simulink model "test_lqi"  (R2018b)
settings: Solver=VariableStepAuto  StartTime=0.0  StopTime=50  RelTol=1e-3
values from neighbouring files (symbols this model uses):
  A = [ 0 0 1 0 ... (first row only)    [ControlParameters.m]    (also in FrutaFuruta.m; furutadynamics.m)
  B1 = [0; 0 ; b31 ; b41]/1000    [ControlParameters.m]    (also in FrutaFuruta.m; furutadynamics.m)
  C = [ 1 0 0 0]    [ControlParameters.m]    (also in FrutaFuruta.m; furutadynamics.m)
  ki = K(5)    [ControlParameters.m]    (also in FrutaFuruta.m; furutadynamics.m)
undefined symbols (not defined in the file or in its folder): K1
settings Model: Creator=Jones  LastModifiedBy=Jones

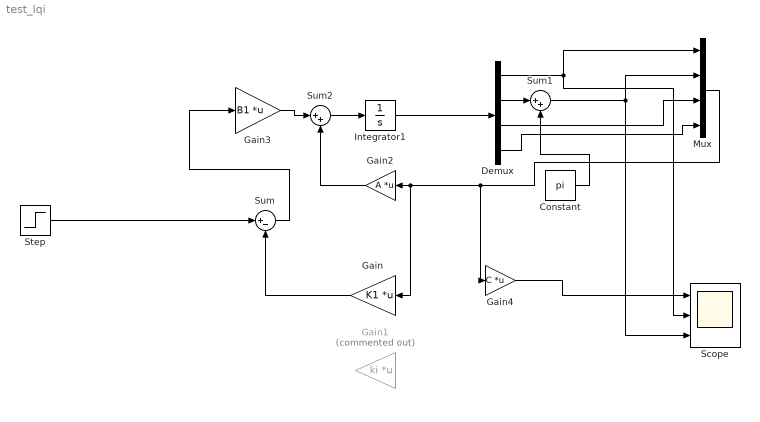
== system test_lqi ==
  Constant : Constant  Value=pi
  Demux : Demux
  Gain : Gain  Gain=K1  Multiplication=Matrix(K*u)
  Gain1 : Gain  Commented=on  Gain=ki  Multiplication=Matrix(K*u)
  Gain2 : Gain  Gain=A  Multiplication=Matrix(K*u)
  Gain3 : Gain  Gain=B1  Multiplication=Matrix(K*u)
  Gain4 : Gain  Gain=C  Multiplication=Matrix(K*u)
  Integrator1 : Integrator
  Mux : Mux
  Scope : Scope  NumInputPorts=3
  Step : Step  Time=0  After=2  SampleTime=0
  Sum : Sum  Inputs=|+-
  Sum1 : Sum  Inputs=|++
  Sum2 : Sum  Inputs=|++
  wires:
  Gain/1 -> Sum/2
  Step/1 -> Sum/1
  Integrator1/1 -> Demux/1
  Sum2/1 -> Integrator1/1
  Gain3/1 -> Sum2/1
  Gain2/1 -> Sum2/2
  Sum/1 -> Gain3/1
  Gain4/1 -> Scope/1
  Constant/1 -> Sum1/2
  Demux/2 -> Sum1/1
  Sum1/1 -> Scope/3, Mux/2
  Demux/1 -> Scope/2, Mux/1
  Demux/3 -> Mux/3
  Demux/4 -> Mux/4
  Mux/1 -> Gain4/1, Gain/1, Gain2/1
